simulink model "Copy_of_ADRC_D_2nd"  (R2022b)
settings: Solver=ode4  StartTime=0.0  StopTime=15  FixedStep=0.001  RelTol=1e-3
settings Model: Creator=玖辞丶  LastModifiedBy=12854
settings SolverCC: AlgebraicLoopSolver=TrustRegion
settings DataIOCC: ReturnWorkspaceOutputs=off
settings DebuggingCC: UnconnectedInputMsg=warning  UnconnectedOutputMsg=warning  UnconnectedLineMsg=warning  SFMachineParentedDataDiag=warning  ArithmeticOperatorsInVariantConditions=warning
settings ModelReferenceCC: EnableRefExpFcnMdlSchedulingChecks=on
settings SFSimCC: CustomCodeUndefinedFunction=UseInterfaceOnly

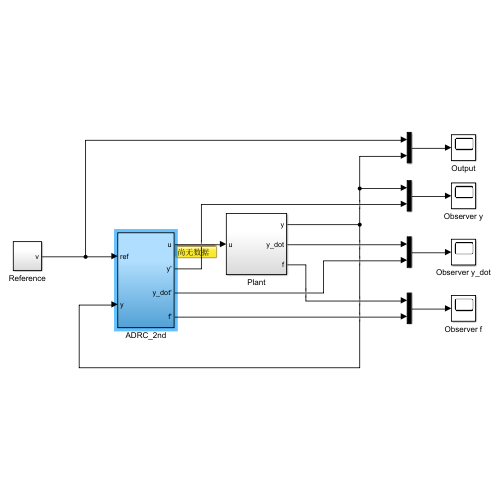
[thumbnail: Simulink's stored preview of the top-level diagram]
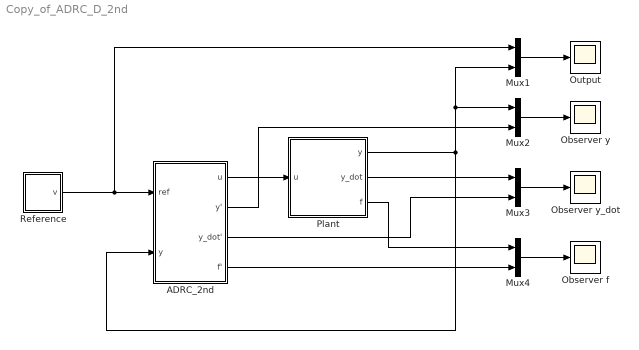
== system Copy_of_ADRC_D_2nd ==
  ADRC_2nd : Subsystem
  Mux{1..4} (4 alike) : Mux  Inputs=2
  Observer f : Scope
  Observer y : Scope
  Observer y_dot : Scope
  Output : Scope
  Plant : Subsystem
  Reference : Subsystem
  wires:
  Reference/1(v) -> Mux1/1, ADRC_2nd/1(ref)
  ADRC_2nd/1(u) -> Plant/1(u)
  Plant/1(y) -> Mux2/1, Mux1/2, ADRC_2nd/2(y)
  Mux1/1 -> Output/1
  Mux2/1 -> Observer y/1
  ADRC_2nd/2(y') -> Mux2/2
  Plant/2(y_dot) -> Mux3/1
  Mux3/1 -> Observer y_dot/1
  Mux4/1 -> Observer f/1
  ADRC_2nd/3(y_dot') -> Mux3/2
  Plant/3(f) -> Mux4/1
  ADRC_2nd/4(f') -> Mux4/2

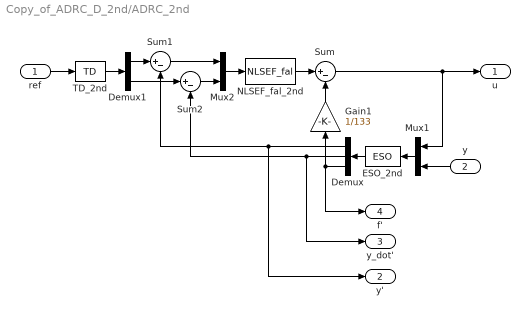
== system Copy_of_ADRC_D_2nd/ADRC_2nd ==
  ref : Inport
  y : Inport  Port=2
  Demux : Demux  Outputs=3
  Demux1 : Demux  Outputs=2
  ESO_2nd : S-Function  FunctionName=ESO  Parameters=CtrlPara  SFunctionDeploymentMode=off  EnableBusSupport=off
  Gain1 : Gain  Gain=1/133
  Mux1 : Mux  Inputs=2
  Mux2 : Mux  Inputs=2
  NLSEF_fal_2nd : S-Function  FunctionName=NLSEF_fal  Parameters=CtrlPara  SFunctionDeploymentMode=off  EnableBusSupport=off
  Sum : Sum  Inputs=|+-
  Sum1 : Sum  Inputs=|+-
  Sum2 : Sum  Inputs=|+-
  TD_2nd : S-Function  FunctionName=TD  Parameters=CtrlPara  SFunctionDeploymentMode=off  EnableBusSupport=off
  u : Outport  VectorParamsAs1DForOutWhenUnconnected=off
  y' : Outport  Port=2  VectorParamsAs1DForOutWhenUnconnected=off
  y_dot' : Outport  Port=3  VectorParamsAs1DForOutWhenUnconnected=off
  f' : Outport  Port=4  VectorParamsAs1DForOutWhenUnconnected=off
  wires:
  Mux2/1 -> NLSEF_fal_2nd/1
  ESO_2nd/1 -> Demux/1
  Demux1/2 -> Sum2/1
  ref/1 -> TD_2nd/1
  Demux/1 -> y'/1, Sum1/2
  TD_2nd/1 -> Demux1/1
  y/1 -> Mux1/2
  Gain1/1 -> Sum/2
  Demux/2 -> y_dot'/1, Sum2/2
  Demux1/1 -> Sum1/1
  Demux/3 -> Gain1/1, f'/1
  Sum2/1 -> Mux2/2
  Sum/1 -> Mux1/1, u/1
  NLSEF_fal_2nd/1 -> Sum/1
  Sum1/1 -> Mux2/1
  Mux1/1 -> ESO_2nd/1

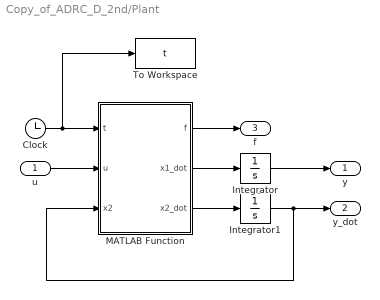
== system Copy_of_ADRC_D_2nd/Plant ==
  u : Inport
  Clock : Clock
  Integrator : Integrator
  Integrator1 : Integrator
  MATLAB Function : MATLAB Function  TreatAsAtomicUnit=on
  To Workspace : ToWorkspace  VariableName=t  SampleTime=-1
  y : Outport  VectorParamsAs1DForOutWhenUnconnected=off
  y_dot : Outport  Port=2  VectorParamsAs1DForOutWhenUnconnected=off
  f : Outport  Port=3  VectorParamsAs1DForOutWhenUnconnected=off
  wires:
  u/1 -> MATLAB Function/2(u)
  MATLAB Function/2(x1_dot) -> Integrator/1
  MATLAB Function/1(f) -> f/1
  Integrator1/1 -> MATLAB Function/3(x2), y_dot/1
  MATLAB Function/3(x2_dot) -> Integrator1/1
  Integrator/1 -> y/1
  Clock/1 -> To Workspace/1, MATLAB Function/1(t)

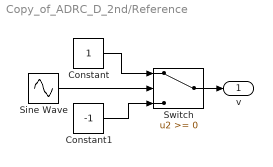
== system Copy_of_ADRC_D_2nd/Reference ==
  Constant : Constant
  Constant1 : Constant  Value=-1
  Sine Wave : Sin  Frequency=0.75  SampleTime=0
  Switch : Switch  SaturateOnIntegerOverflow=off  InputSameDT=off
  v : Outport  VectorParamsAs1DForOutWhenUnconnected=off
  wires:
  Constant1/1 -> Switch/3
  Sine Wave/1 -> Switch/2
  Constant/1 -> Switch/1
  Switch/1 -> v/1

== matlab function Copy_of_ADRC_D_2nd/Plant/MATLAB Function ==
  data: f output; t input; u input; x2 input; x1_dot output; x2_dot output
function [f, x1_dot, x2_dot] = fcn(t, u, x2)

x1_dot = x2;
x2_dot = -25 * x2 + 33 * sin(pi*t) + 133 * u;
f = -25 * x2 + 33 * sin(pi*t);
end
